simulink model "ifaction_task"  (R2021a)
settings: Solver=VariableStepAuto  StartTime=0.0  StopTime=10.0  RelTol=1e-3
libraries: simulink x1
settings Model: Creator=reemb  LastModifiedBy=reemb

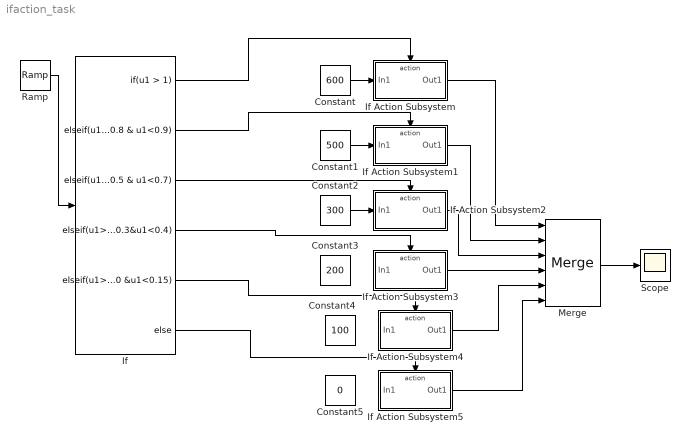
== system ifaction_task ==
  Constant : Constant  Value=600
  Constant1 : Constant  Value=500
  Constant2 : Constant  Value=300
  Constant3 : Constant  Value=200
  Constant4 : Constant  Value=100
  Constant5 : Constant  Value=0
  If : If  IfExpression=u1 > 1  ElseIfExpressions="u1>0.8 & u1<0.9 , u1>0.5 & u1<0.7  ,   u1>0.3&u1<0.4   ,   u1>0 &u1<0.15"
  If Action Subsystem : Subsystem  TreatAsAtomicUnit=on
  If Action Subsystem1 : Subsystem  TreatAsAtomicUnit=on
  If Action Subsystem2 : Subsystem  TreatAsAtomicUnit=on
  If Action Subsystem3 : Subsystem  TreatAsAtomicUnit=on
  If Action Subsystem4 : Subsystem  TreatAsAtomicUnit=on
  If Action Subsystem5 : Subsystem  TreatAsAtomicUnit=on
  Merge : Merge  Inputs=6
  Ramp : simulink/Sources/Ramp  slope=1  start=0  InitialOutput=0
  Scope : Scope
  wires:
  Ramp/1 -> If/1
  Constant/1 -> If Action Subsystem/1(In1)
  Constant1/1 -> If Action Subsystem1/1(In1)
  Constant2/1 -> If Action Subsystem2/1(In1)
  Merge/1 -> Scope/1
  If Action Subsystem/1(Out1) -> Merge/1
  If Action Subsystem1/1(Out1) -> Merge/2
  If Action Subsystem2/1(Out1) -> Merge/3
  If Action Subsystem3/1(Out1) -> Merge/4
  If Action Subsystem4/1(Out1) -> Merge/5
  If Action Subsystem5/1(Out1) -> Merge/6
  If/1 -> If Action Subsystem/Action
  If/2 -> If Action Subsystem1/Action
  If/3 -> If Action Subsystem2/Action
  If/4 -> If Action Subsystem3/Action
  If/5 -> If Action Subsystem4/Action
  If/6 -> If Action Subsystem5/Action

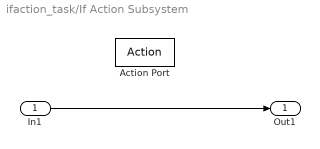
== system ifaction_task/If Action Subsystem ==
  In1 : Inport
  Action Port : ActionPort  ActionPortLabel=if(u1 > 1)
  Out1 : Outport
  wires:
  In1/1 -> Out1/1

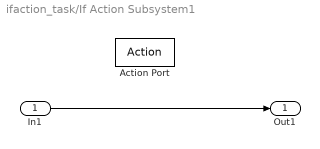
== system ifaction_task/If Action Subsystem1 ==
  In1 : Inport
  Action Port : ActionPort  ActionPortLabel=elseif(u1>0.8 & u1<0.9 )
  Out1 : Outport
  wires:
  In1/1 -> Out1/1

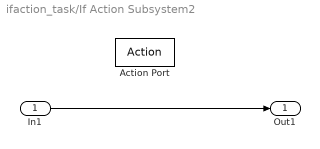
== system ifaction_task/If Action Subsystem2 ==
  In1 : Inport
  Action Port : ActionPort  ActionPortLabel="elseif( u1>0.5 & u1<0.7  )"
  Out1 : Outport
  wires:
  In1/1 -> Out1/1

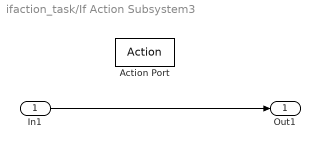
== system ifaction_task/If Action Subsystem3 ==
  In1 : Inport
  Action Port : ActionPort  ActionPortLabel="elseif(   u1>0.3&u1<0.4   )"
  Out1 : Outport
  wires:
  In1/1 -> Out1/1

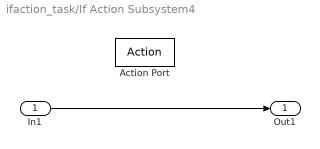
== system ifaction_task/If Action Subsystem4 ==
  In1 : Inport
  Action Port : ActionPort  ActionPortLabel="elseif(   u1>0 &u1<0.15)"
  Out1 : Outport
  wires:
  In1/1 -> Out1/1

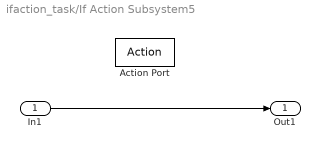
== system ifaction_task/If Action Subsystem5 ==
  In1 : Inport
  Action Port : ActionPort  ActionPortLabel=else
  Out1 : Outport
  wires:
  In1/1 -> Out1/1
